simulink model "MPC_MEMS"  (Simulink 8.5)
settings: Solver=ode5  StartTime=0.0  StopTime=4.99  FixedStep=1e-3  RelTol=1e-3
values from neighbouring files (symbols this model uses):
  A = [Am o4 o4;Cm*Am 2*eye(2) -(1+(w1*dt)^2)*eye(2);o4' eye(2) zeros(2,2)]    [DMPC_MEMS_Gyro.m]
  A_cons = [L_m;-L_m]    [DMPC_MEMS_Gyro.m]
  B = [Bm;Cm*Bm;zeros(2,2)]    [DMPC_MEMS_Gyro.m]
  C = [zeros(2,4) eye(2) zeros(2,2)]    [DMPC_MEMS_Gyro.m]
  dt = 0.001    [DMPC_MEMS_Gyro.m]
  Lf = Kalman_Gain(A,C,Qf,Rf,Pf,Nsim)    [DMPC_MEMS_Gyro.m]
  u_bound = [u_max;-u_min]    [DMPC_MEMS_Gyro.m]
  w1 = 1.191931942010938e+002    (= 119.193194201)    [DMPC_MEMS_Gyro.m]
  x0 = 0.1    [DMPC_MEMS_Gyro.m]
undefined symbols (not defined in the file or in its folder): Ag, Bg, Cg, L_m, omega, psi
settings Model: Creator=Farhang  LastModifiedBy=p4wp4w
settings DebuggingCC: SolverPrmCheckMsg=warning  FcnCallInpInsideContextMsg=UseLocalSettings

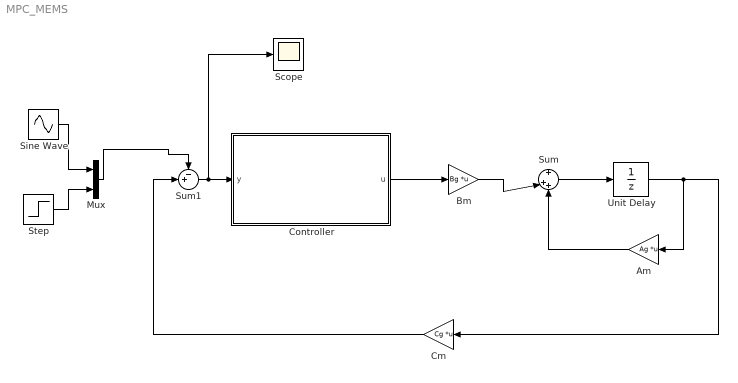
== system MPC_MEMS ==
  Am : Gain  Gain=Ag  Multiplication=Matrix(K*u)
  Bm : Gain  Gain=Bg  Multiplication=Matrix(K*u)
  Cm : Gain  Gain=Cg  Multiplication=Matrix(K*u)
  Controller : Subsystem
  Mux : Mux  Inputs=2
  Scope : Scope
  Sine Wave : Sin  Amplitude=x0  Frequency=w1  SampleTime=0
  Step : Step  Time=0  After=0  SampleTime=0
  Sum : Sum  Inputs=+|++
  Sum1 : Sum  Inputs=-+|
  Unit Delay : UnitDelay  SampleTime=dt
  wires:
  Unit Delay/1 -> Am/1, Cm/1
  Controller/1(u) -> Bm/1
  Am/1 -> Sum/3
  Bm/1 -> Sum/2
  Sum/1 -> Unit Delay/1
  Sine Wave/1 -> Mux/1
  Step/1 -> Mux/2
  Sum1/1 -> Controller/1(y), Scope/1
  Mux/1 -> Sum1/1
  Cm/1 -> Sum1/2

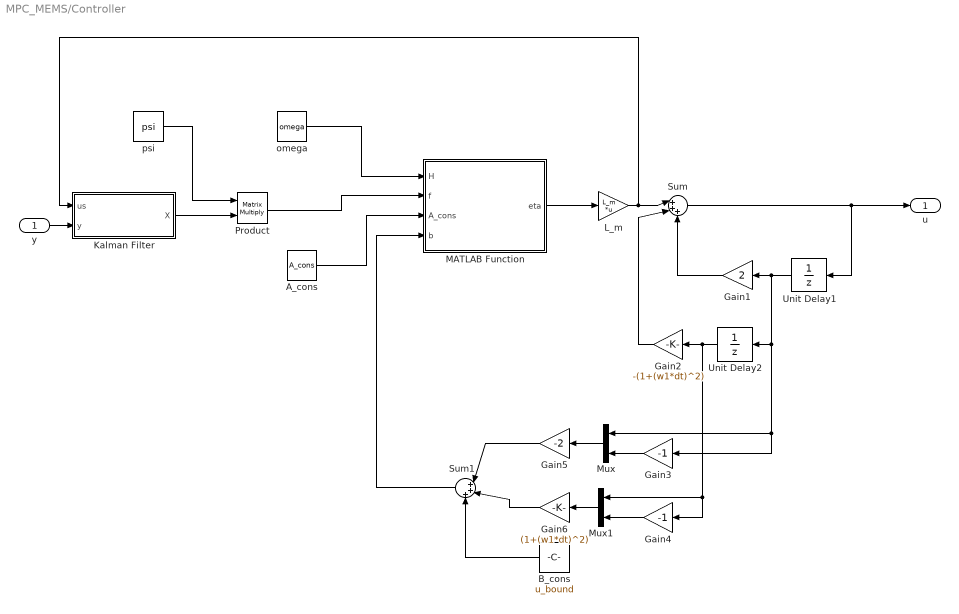
== system MPC_MEMS/Controller ==
  y : Inport
  A_cons : Constant  Value=A_cons
  B_cons : Constant  Value=u_bound
  Gain1 : Gain  Gain=2
  Gain2 : Gain  Gain=-(1+(w1*dt)^2)
  Gain3 : Gain  Gain=-1
  Gain4 : Gain  Gain=-1
  Gain5 : Gain  Gain=-2
  Gain6 : Gain  Gain=(1+(w1*dt)^2)
  Kalman Filter : Subsystem  TreatAsAtomicUnit=on
  L_m : Gain  Gain=L_m  Multiplication=Matrix(K*u)
  MATLAB Function : MATLAB Function  TreatAsAtomicUnit=on
  Mux : Mux  Inputs=2
  Mux1 : Mux  Inputs=2
  Product : Product  Multiplication=Matrix(*)  RndMeth=Zero
  Sum : Sum  Inputs=|+++
  Sum1 : Sum  Inputs=|+++
  Unit Delay1 : UnitDelay  SampleTime=dt
  Unit Delay2 : UnitDelay  SampleTime=dt
  omega : Constant  Value=omega
  psi : Constant  Value=psi
  u : Outport
  wires:
  MATLAB Function/1(eta) -> L_m/1
  L_m/1 -> Sum/1, Kalman Filter/1(us)
  Sum/1 -> Unit Delay1/1, u/1
  Unit Delay1/1 -> Gain1/1, Unit Delay2/1, Mux/1, Gain3/1
  Gain1/1 -> Sum/3
  Unit Delay2/1 -> Gain2/1, Mux1/1, Gain4/1
  Gain2/1 -> Sum/2
  Gain3/1 -> Mux/2
  Gain4/1 -> Mux1/2
  Mux/1 -> Gain5/1
  Gain5/1 -> Sum1/1
  Mux1/1 -> Gain6/1
  Gain6/1 -> Sum1/2
  B_cons/1 -> Sum1/3
  Sum1/1 -> MATLAB Function/4(b)
  omega/1 -> MATLAB Function/1(H)
  A_cons/1 -> MATLAB Function/3(A_cons)
  psi/1 -> Product/1
  Kalman Filter/1(X) -> Product/2
  Product/1 -> MATLAB Function/2(f)
  y/1 -> Kalman Filter/2(y)

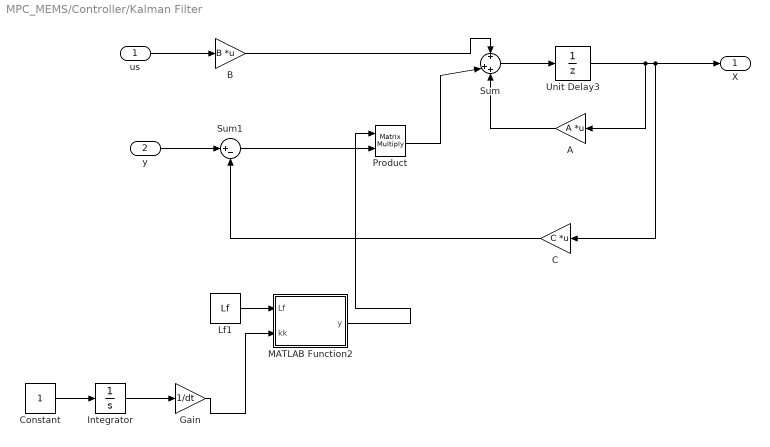
== system MPC_MEMS/Controller/Kalman Filter ==
  us : Inport
  y : Inport  Port=2
  A : Gain  Gain=A  Multiplication=Matrix(K*u)
  B : Gain  Gain=B  Multiplication=Matrix(K*u)
  C : Gain  Gain=C  Multiplication=Matrix(K*u)
  Constant : Constant
  Gain : Gain  Gain=1/dt
  Integrator : Integrator
  Lf1 : Constant  Value=Lf
  MATLAB Function2 : MATLAB Function  TreatAsAtomicUnit=on
  Product : Product  Multiplication=Matrix(*)  RndMeth=Zero
  Sum : Sum  Inputs=+|++
  Sum1 : Sum  Inputs=|+-
  Unit Delay3 : UnitDelay  SampleTime=dt
  X : Outport
  wires:
  Unit Delay3/1 -> A/1, X/1, C/1
  A/1 -> Sum/3
  Sum/1 -> Unit Delay3/1
  us/1 -> B/1
  B/1 -> Sum/1
  C/1 -> Sum1/2
  y/1 -> Sum1/1
  Sum1/1 -> Product/2
  Product/1 -> Sum/2
  Constant/1 -> Integrator/1
  Integrator/1 -> Gain/1
  Lf1/1 -> MATLAB Function2/1(Lf)
  Gain/1 -> MATLAB Function2/2(kk)
  MATLAB Function2/1(y) -> Product/1

== matlab function Controller/MATLAB Function ==
  data: H input double; eta output double; f input double; A_cons input double; b input double
function eta=QPhild(H,f,A_cons,b)
% E=H;
% F=f;
% M=A_cons;
% gamma=b;
% eta =x
[n1,m1]=size(A_cons);
eta=-H\f;
kk=0;
for i=1:n1
if (A_cons(i,:)*eta>b(i)) 
    kk=kk+1;
else
kk=kk+0;
end
end
if (kk==0)
    return
end
P=A_cons*(H\A_cons');
d=(A_cons*(H\f)+b);
[n,m]=size(d);
x_ini=zeros(n,m);
lambda=x_ini;
al=10;
for km=1:38
%find the elements in the solution vector one by one
% km could be larger if the Lagranger multiplier has a slow
% convergence rate.
lambda_p=lambda;
for i=1:n
w= P(i,:)*lambda-P(i,i)*lambda(i,1);
w=w+d(i,1);
la=-w/P(i,i);
lambda(i,1)=max(0,la);
end
al=(lambda-lambda_p)'*(lambda-lambda_p);
if (al<10e-8); break; end
end
eta=-H\f -H\A_cons'*lambda;

== matlab function Controller/Kalman Filter/MATLAB Function2 ==
  data: y output double; Lf input double; kk input double
function y = fcn(Lf,kk)
%#codegen

kk = floor(kk)+1;

y = Lf(:,2*kk-1:2*kk);
